simulink model "snb_b_ser2par"  (R2012b)
(part 2 of 57)

      |     current_names = current_names{1};
      |     numios = length(current_names);
      |     if length(current_widths) ~= numios,
      |         error('%d field names specified, but %d widths?', numios, length(current_widths));
      |     end
      | end
      | total_width = 0;
      | for ctr = 1 : length(current_widths),
      |     total_width = total_width + current_widths(ctr);
      | end
      | if total_width > 32,
      |     error('Total width must be 32 or less, set to %d.', total_width);
      | end
      mask Callback arith_types:
      | blk = gcb;
      | mode = get_param(blk, 'mode');
      | current_types = eval(get_param(blk, 'arith_types'));
      | numios = length(current_types);
      | if (strcmp(mode, 'one value') || strcmp(mode, 'fields of equal size')) && (length(current_types) > 1),
      |     error('Only one type may be specified for this mode.');
      | elseif strcmp(mode, 'fields of arbitrary size')
      |     current_names = textscan(strtrim(strrep(strrep(get_param(blk, 'names'), ']', ''), '[', '')), '%s');
      |     current_names = current_names{1};
      |     numios = length(current_names);
      |     if length(current_types) ~= numios,
      |         error('%d field names specified, but %d types?', numios, length(current_types));
      |     end
      | end
      | problem = 0;
      | for ctr = 1 : numios,
      |     t = current_types(ctr);
      |     if (t < 0) || (t > 2),
      |         problem = t;
      |         ctr = numios + 1;
      |     end
      | end
      | if problem ~= 0,
      |     error('Type cannot be %i, must be 0, 1 or 2.', problem);
      | end
      mask Callback bin_pts:
      | blk = gcb;
      | mode = get_param(blk, 'mode');
      | current_bins = eval(get_param(blk, 'bin_pts'));
      | if (strcmp(mode, 'one value') || strcmp(mode, 'fields of equal size')) && (length(current_bins) > 1),
      |     error('Only one binary pt may be specified for this mode.');
      | elseif strcmp(mode, 'fields of arbitrary size')
      |     current_names = textscan(strtrim(strrep(strrep(get_param(blk, 'names'), ']', ''), '[', '')), '%s');
      |     current_names = current_names{1};
      |     numios = length(current_names);
      |     if length(current_bins) ~= numios,
      |         error('%d field names specified, but %d binary pts?', numios, length(current_bins));
      |     end
      | end
  tmiss_p1 : Subsystem  Tag=xps:sw_reg  AncestorBlock=xps_library/software register  mask(swreg){mode=one value, io_dir=To Processor, io_delay=0, sample_period=1, names=reg, bitwidths=32, arith_types=0, bin_pts=0, sim_port=off, show_format=on}
      mask prompts: io_dir "I/O direction"; io_delay "I/O delay"; sample_period "Sample period"; names "Name:"; bitwidths "Bitwidth:"; arith_types "Type (ufix=0, fix=1, bool=2):"; bin_pts "Binary pt:"; sim_port "Provide sim input/output?"; show_format "Print format string?"
      mask init:
      | swreg_init(gcb)
      settings: AttributesFormatString=1output:uf32.0,
      mask TypeOptions mode: one value | fields of equal size | fields of arbitrary size
      mask Callback mode: swreg_cb(gcb);
      mask TypeOptions io_dir: To Processor | From Processor
      mask Callback io_dir:
      | mask_enables = get_param(gcb, 'MaskEnables');
      | mask_names = get_param(gcb, 'MaskNames');
      | if strcmp(get_param(gcb, 'io_dir'), 'To Processor'),
      |     mask_enables{ismember(mask_names, 'sample_period')} = 'off';
      | else
      |     mask_enables{ismember(mask_names, 'sample_period')} = 'on';
      | end
      | set_param(gcb, 'MaskEnables', mask_enables);
      mask Callback bitwidths:
      | blk = gcb;
      | mode = get_param(blk, 'mode');
      | current_widths = eval(get_param(blk, 'bitwidths'));
      | if (strcmp(mode, 'one value') || strcmp(mode, 'fields of equal size')) && (length(current_widths) > 1),
      |     error('Only one width may be specified for this mode.');
      | elseif strcmp(mode, 'fields of arbitrary size')
      |     current_names = textscan(strtrim(strrep(strrep(get_param(blk, 'names'), ']', ''), '[', '')), '%s');
      |     current_names = current_names{1};
      |     numios = length(current_names);
      |     if length(current_widths) ~= numios,
      |         error('%d field names specified, but %d widths?', numios, length(current_widths));
      |     end
      | end
      | total_width = 0;
      | for ctr = 1 : length(current_widths),
      |     total_width = total_width + current_widths(ctr);
      | end
      | if total_width > 32,
      |     error('Total width must be 32 or less, set to %d.', total_width);
      | end
      mask Callback arith_types:
      | blk = gcb;
      | mode = get_param(blk, 'mode');
      | current_types = eval(get_param(blk, 'arith_types'));
      | numios = length(current_types);
      | if (strcmp(mode, 'one value') || strcmp(mode, 'fields of equal size')) && (length(current_types) > 1),
      |     error('Only one type may be specified for this mode.');
      | elseif strcmp(mode, 'fields of arbitrary size')
      |     current_names = textscan(strtrim(strrep(strrep(get_param(blk, 'names'), ']', ''), '[', '')), '%s');
      |     current_names = current_names{1};
      |     numios = length(current_names);
      |     if length(current_types) ~= numios,
      |         error('%d field names specified, but %d types?', numios, length(current_types));
      |     end
      | end
      | problem = 0;
      | for ctr = 1 : numios,
      |     t = current_types(ctr);
      |     if (t < 0) || (t > 2),
      |         problem = t;
      |         ctr = numios + 1;
      |     end
      | end
      | if problem ~= 0,
      |     error('Type cannot be %i, must be 0, 1 or 2.', problem);
      | end
      mask Callback bin_pts:
      | blk = gcb;
      | mode = get_param(blk, 'mode');
      | current_bins = eval(get_param(blk, 'bin_pts'));
      | if (strcmp(mode, 'one value') || strcmp(mode, 'fields of equal size')) && (length(current_bins) > 1),
      |     error('Only one binary pt may be specified for this mode.');
      | elseif strcmp(mode, 'fields of arbitrary size')
      |     current_names = textscan(strtrim(strrep(strrep(get_param(blk, 'names'), ']', ''), '[', '')), '%s');
      |     current_names = current_names{1};
      |     numios = length(current_names);
      |     if length(current_bins) ~= numios,
      |         error('%d field names specified, but %d binary pts?', numios, length(current_bins));
      |     end
      | end
  trig0 : Subsystem  mask{mult_latency=3}
      mask prompts: mult_latency "Multiplier latency"
  trig1 : Subsystem  mask{mult_latency=3}
      mask prompts: mult_latency "Multiplier latency"
  trigger_level : Subsystem  Tag=xps:sw_reg  AncestorBlock=xps_library/software register  mask(swreg){mode=one value, io_dir=From Processor, io_delay=0, sample_period=1, names=trigger_level, bitwidths=32, arith_types=0, bin_pts=0, show_format=off}
      mask prompts: io_dir "I/O direction"; io_delay "I/O delay"; sample_period "Sample period"; names "Name:"; bitwidths "Bitwidth:"; arith_types "Type (ufix=0, fix=1, bool=2):"; bin_pts "Binary pt:"; show_format "Print format string?"
      mask init:
      | swreg_init(gcb)
      settings: AttributesFormatString=1input
      mask TypeOptions mode: one value | fields of equal size | fields of arbitrary size
      mask Callback mode: swreg_cb(gcb);
      mask TypeOptions io_dir: To Processor | From Processor
      mask Callback io_dir:
      | mask_enables = get_param(gcb, 'MaskEnables');
      | mask_names = get_param(gcb, 'MaskNames');
      | if strcmp(get_param(gcb, 'io_dir'), 'To Processor'),
      |     mask_enables{ismember(mask_names, 'sample_period')} = 'off';
      | else
      |     mask_enables{ismember(mask_names, 'sample_period')} = 'on';
      | end
      | set_param(gcb, 'MaskEnables', mask_enables);
      mask Callback bitwidths:
      | blk = gcb;
      | mode = get_param(blk, 'mode');
      | current_widths = eval(get_param(blk, 'bitwidths'));
      | if (strcmp(mode, 'one value') || strcmp(mode, 'fields of equal size')) && (length(current_widths) > 1),
      |     error('Only one width may be specified for this mode.');
      | elseif strcmp(mode, 'fields of arbitrary size')
      |     current_names = textscan(strtrim(strrep(strrep(get_param(blk, 'names'), ']', ''), '[', '')), '%s');
      |     current_names = current_names{1};
      |     numios = length(current_names);
      |     if length(current_widths) ~= numios,
      |         error('%d field names specified, but %d widths?', numios, length(current_widths));
      |     end
      | end
      | total_width = 0;
      | for ctr = 1 : length(current_widths),
      |     total_width = total_width + current_widths(ctr);
      | end
      | if total_width > 32,
      |     error('Total width must be 32 or less, set to %d.', total_width);
      | end
      mask Callback arith_types:
      | blk = gcb;
      | mode = get_param(blk, 'mode');
      | current_types = eval(get_param(blk, 'arith_types'));
      | numios = length(current_types);
      | if (strcmp(mode, 'one value') || strcmp(mode, 'fields of equal size')) && (length(current_types) > 1),
      |     error('Only one type may be specified for this mode.');
      | elseif strcmp(mode, 'fields of arbitrary size')
      |     current_names = textscan(strtrim(strrep(strrep(get_param(blk, 'names'), ']', ''), '[', '')), '%s');
      |     current_names = current_names{1};
      |     numios = length(current_names);
      |     if length(current_types) ~= numios,
      |         error('%d field names specified, but %d types?', numios, length(current_types));
      |     end
      | end
      | problem = 0;
      | for ctr = 1 : numios,
      |     t = current_types(ctr);
      |     if (t < 0) || (t > 2),
      |         problem = t;
      |         ctr = numios + 1;
      |     end
      | end
      | if problem ~= 0,
      |     error('Type cannot be %i, must be 0, 1 or 2.', problem);
      | end
      mask Callback bin_pts:
      | blk = gcb;
      | mode = get_param(blk, 'mode');
      | current_bins = eval(get_param(blk, 'bin_pts'));
      | if (strcmp(mode, 'one value') || strcmp(mode, 'fields of equal size')) && (length(current_bins) > 1),
      |     error('Only one binary pt may be specified for this mode.');
      | elseif strcmp(mode, 'fields of arbitrary size')
      |     current_names = textscan(strtrim(strrep(strrep(get_param(blk, 'names'), ']', ''), '[', '')), '%s');
      |     current_names = current_names{1};
      |     numios = length(current_names);
      |     if length(current_bins) ~= numios,
      |         error('%d field names specified, but %d binary pts?', numios, length(current_bins));
      |     end
      | end
  tx_metadata : Subsystem  Tag=xps:sw_reg  AncestorBlock=xps_library/software register  mask(swreg){mode=fields of arbitrary size, io_dir=From Processor, io_delay=0, sample_period=1, names=[porttx board_id], bitwidths=16, arith_types=0, bin_pts=0, sim_port=on, show_format=off}
      mask prompts: io_dir "I/O direction"; io_delay "I/O delay"; sample_period "Sample period"; names "Names [msb ... lsb]:"; bitwidths "Bitwidths [msb ... lsb]:"; arith_types "Types (ufix=0, fix=1, bool=2) [msb ... lsb]:"; bin_pts "Binary pts [msb ... lsb]:"; sim_port "Provide sim input/output?"; show_format "Print format string?"
      mask init:
      | swreg_init(gcb)
      settings: AttributesFormatString=2 inputs
      mask TypeOptions mode: one value | fields of equal size | fields of arbitrary size
      mask Callback mode: swreg_cb(gcb);
      mask TypeOptions io_dir: To Processor | From Processor
      mask Callback io_dir:
      | mask_enables = get_param(gcb, 'MaskEnables');
      | mask_names = get_param(gcb, 'MaskNames');
      | if strcmp(get_param(gcb, 'io_dir'), 'To Processor'),
      |     mask_enables{ismember(mask_names, 'sample_period')} = 'off';
      | else
      |     mask_enables{ismember(mask_names, 'sample_period')} = 'on';
      | end
      | set_param(gcb, 'MaskEnables', mask_enables);
      mask Callback bitwidths:
      | swreg_maskcheck(gcb);
      | % blk = gcb;
      | % mode = get_param(blk, 'mode');
      | % current_widths = eval(get_param(blk, 'bitwidths'));
      | % if (strcmp(mode, 'one value') || strcmp(mode, 'fields of equal size')) && (length(current_widths) > 1),
      | %     error('Only one width may be specified for this mode.');
      | % elseif strcmp(mode, 'fields of arbitrary size')
      | %     current_names = textscan(strtrim(strrep(strrep(get_param(blk, 'names'), ']', ''), '[', '')), '%s');
      | %     current_names = current_names{1};
      | %     numios = length(current_names);
      | %     if length(current_widths) ~= numios,
      | %         error('%d field names specified, but %d widths?', numios, length(current_widths));
      | %     end
      | % end
      | % total_width = 0;
      | % for ctr = 1 : length(current_widths),
      | %     total_width = total_width + current_widths(ctr);
      | % end
      | % if total_width > 32,
      | %     error('Total width must be 32 or less, set to %d.', total_width);
      | % end
      mask Callback arith_types:
      | [numios, ~, ~, ~, current_types] = swreg_maskcheck(gcb);
      | % blk = gcb;
      | % mode = get_param(blk, 'mode');
      | % current_types = eval(get_param(blk, 'arith_types'));
      | % numios = length(current_types);
      | % if (strcmp(mode, 'one value') || strcmp(mode, 'fields of equal size')) && (length(current_types) > 1),
      | %     error('Only one type may be specified for this mode.');
      | % elseif strcmp(mode, 'fields of arbitrary size')
      | %     current_names = textscan(strtrim(strrep(strrep(get_param(blk, 'names'), ']', ''), '[', '')), '%s');
      | %     current_names = current_names{1};
      | %     numios = length(current_names);
      | %     if length(current_types) ~= numios,
      | %         error('%d field names specified, but %d types?', numios, length(current_types));
      | %     end
      | % end
      | problem = 0;
      | for ctr = 1 : numios,
      |     t = current_types(ctr);
      |     if (t < 0) || (t > 2),
      |         problem = t;
      |         ctr = numios + 1;
      |     end
      | end
      | if problem ~= 0,
      |     error('Type cannot be %i, must be 0, 1 or 2.', problem);
      | end
      mask Callback bin_pts:
      | swreg_maskcheck(gcb);
      | % blk = gcb;
      | % mode = get_param(blk, 'mode');
      | % current_bins = eval(get_param(blk, 'bin_pts'));
      | % if (strcmp(mode, 'one value') || strcmp(mode, 'fields of equal size')) && (length(current_bins) > 1),
      | %     error('Only one binary pt may be specified for this mode.');
      | % elseif strcmp(mode, 'fields of arbitrary size')
      | %     current_names = textscan(strtrim(strrep(strrep(get_param(blk, 'names'), ']', ''), '[', '')), '%s');
      | %     current_names = current_names{1};
      | %     numios = length(current_names);
      | %     if length(current_bins) ~= numios,
      | %         error('%d field names specified, but %d binary pts?', numios, length(current_bins));
      | %     end
      | % end
  unpack_and_reorder : Subsystem  mask{n_bits_packet_size=9, n_bits_timestep=9+3, n_bits_fifo_depth=3, n_bits_buffer_depth=3, bram_latency=1}
      mask prompts: n_bits_packet_size "Packet size (2^? 80-bit words after unpacking)"; n_bits_timestep "Packet timestep (2^?)"; n_bits_fifo_depth "FIFO depth (2^? packets)"; n_bits_buffer_depth "Reorder buffer size (2^? packets)"; bram_latency "BRAM latency"
  up_debug : Subsystem  Tag=xps:sw_reg  AncestorBlock=xps_library/software register  mask(swreg){mode=one value, io_dir=From Processor, io_delay=0, sample_period=1, names=gbe_timestep, bitwidths=3, arith_types=0, bin_pts=0, sim_port=off, show_format=on}
      mask prompts: io_dir "I/O direction"; io_delay "I/O delay"; sample_period "Sample period"; names "Name:"; bitwidths "Bitwidth:"; arith_types "Type (ufix=0, fix=1, bool=2):"; bin_pts "Binary pt:"; sim_port "Provide sim input/output?"; show_format "Print format string?"
      mask init:
      | swreg_init(gcb)
      settings: AttributesFormatString=1input:uf3.0,
      mask TypeOptions mode: one value | fields of equal size | fields of arbitrary size
      mask Callback mode: swreg_cb(gcb);
      mask TypeOptions io_dir: To Processor | From Processor
      mask Callback io_dir:
      | mask_enables = get_param(gcb, 'MaskEnables');
      | mask_names = get_param(gcb, 'MaskNames');
      | if strcmp(get_param(gcb, 'io_dir'), 'To Processor'),
      |     mask_enables{ismember(mask_names, 'sample_period')} = 'off';
      | else
      |     mask_enables{ismember(mask_names, 'sample_period')} = 'on';
      | end
      | set_param(gcb, 'MaskEnables', mask_enables);
      mask Callback bitwidths:
      | blk = gcb;
      | mode = get_param(blk, 'mode');
      | current_widths = eval(get_param(blk, 'bitwidths'));
      | if (strcmp(mode, 'one value') || strcmp(mode, 'fields of equal size')) && (length(current_widths) > 1),
      |     error('Only one width may be specified for this mode.');
      | elseif strcmp(mode, 'fields of arbitrary size')
      |     current_names = textscan(strtrim(strrep(strrep(get_param(blk, 'names'), ']', ''), '[', '')), '%s');
      |     current_names = current_names{1};
      |     numios = length(current_names);
      |     if length(current_widths) ~= numios,
      |         error('%d field names specified, but %d widths?', numios, length(current_widths));
      |     end
      | end
      | total_width = 0;
      | for ctr = 1 : length(current_widths),
      |     total_width = total_width + current_widths(ctr);
      | end
      | if total_width > 32,
      |     error('Total width must be 32 or less, set to %d.', total_width);
      | end
      mask Callback arith_types:
      | blk = gcb;
      | mode = get_param(blk, 'mode');
      | current_types = eval(get_param(blk, 'arith_types'));
      | numios = length(current_types);
      | if (strcmp(mode, 'one value') || strcmp(mode, 'fields of equal size')) && (length(current_types) > 1),
      |     error('Only one type may be specified for this mode.');
      | elseif strcmp(mode, 'fields of arbitrary size')
      |     current_names = textscan(strtrim(strrep(strrep(get_param(blk, 'names'), ']', ''), '[', '')), '%s');
      |     current_names = current_names{1};
      |     numios = length(current_names);
      |     if length(current_types) ~= numios,
      |         error('%d field names specified, but %d types?', numios, length(current_types));
      |     end
      | end
      | problem = 0;
      | for ctr = 1 : numios,
      |     t = current_types(ctr);
      |     if (t < 0) || (t > 2),
      |         problem = t;
      |         ctr = numios + 1;
      |     end
      | end
      | if problem ~= 0,
      |     error('Type cannot be %i, must be 0, 1 or 2.', problem);
      | end
      mask Callback bin_pts:
      | blk = gcb;
      | mode = get_param(blk, 'mode');
      | current_bins = eval(get_param(blk, 'bin_pts'));
      | if (strcmp(mode, 'one value') || strcmp(mode, 'fields of equal size')) && (length(current_bins) > 1),
      |     error('Only one binary pt may be specified for this mode.');
      | elseif strcmp(mode, 'fields of arbitrary size')
      |     current_names = textscan(strtrim(strrep(strrep(get_param(blk, 'names'), ']', ''), '[', '')), '%s');
      |     current_names = current_names{1};
      |     numios = length(current_names);
      |     if length(current_bins) ~= numios,
      |         error('%d field names specified, but %d binary pts?', numios, length(current_bins));
      |     end
      | end
  updebug : Subsystem
      mask Display: fprintf('UP\nDEBUG')
  xps : xps_library/XSG core config  Tag=xps:xsg  hw_sys=ROACH2:sx475t  clk_src=sys_clk  ROACH_clk_src=adc0_clk  ROACH2_clk_src=sys_clk  MKDIG_clk_src=sys_clk  clk_rate=228  sample_period=1  synthesis_tool=XST
  tag scope: cnt_rst=global, gbe_timestep=global, up_cnt_rst=global, wintime_snap_wesel=global
  wires:
  gbe0/1(led_up) -> Inverter/1, [up_gbe0]
  gbe0/2(led_rx) -> [rx_gbe0]
  gbe0/3(led_tx) -> [tx_gbe0]
  gbe0/5(tx_overflow) -> [tx_over_gbe0], [of_xaui0]
  gbe0/12(rx_overrun) -> [rxover_gbe0]
  gbe0/11(rx_bad_frame) -> [rxbad_gbe0]
  gbe0/6(rx_data) -> [rxdata_gbe0]
  gbe0/7(rx_valid) -> [rxvld_gbe0]
  gbe0/8(rx_source_ip) -> [rxip_gbe0]
  gbe0/9(rx_source_port) -> [rxport_gbe0]
  gbe0/10(rx_end_of_frame) -> [rxeof_gbe0]
  Inverter/1 -> [ldn_xaui0]
  [gbe_rst] -> Delay12/1
  gbe1/1(led_up) -> [up_gbe1], Inverter1/1
  gbe1/2(led_rx) -> [rx_gbe1]
  gbe1/3(led_tx) -> [tx_gbe1]
  gbe1/4(tx_afull) -> [tx_full_gbe1]
  gbe1/5(tx_overflow) -> [tx_over_gbe1], [of_xaui1]
  gbe1/12(rx_overrun) -> [rxover_gbe1]
  gbe1/11(rx_bad_frame) -> [rxbad_gbe1]
  gbe1/6(rx_data) -> [rxdata_gbe1]
  gbe1/7(rx_valid) -> [rxvld_gbe1]
  gbe1/8(rx_source_ip) -> [rxip_gbe1]
  gbe1/9(rx_source_port) -> [rxport_gbe1]
  gbe1/10(rx_end_of_frame) -> [rxeof_gbe1]
  Inverter1/1 -> [ldn_xaui1]
  Delay12/1 -> gbe1/1(rst)
  gbe2/1(led_up) -> [up_gbe2], Inverter3/1
  gbe2/2(led_rx) -> [rx_gbe2]
  gbe2/3(led_tx) -> [tx_gbe2]
  gbe2/4(tx_afull) -> [tx_full_gbe2]
  gbe2/5(tx_overflow) -> [tx_over_gbe2], [of_xaui2]
  gbe2/12(rx_overrun) -> [rxover_gbe2]
  gbe2/11(rx_bad_frame) -> [rxbad_gbe2]
  gbe2/6(rx_data) -> [rxdata_gbe2]
  gbe2/7(rx_valid) -> [rxvld_gbe2]
  gbe2/8(rx_source_ip) -> [rxip_gbe2]
  gbe2/9(rx_source_port) -> [rxport_gbe2]
  gbe2/10(rx_end_of_frame) -> [rxeof_gbe2]
  Inverter3/1 -> [ldn_xaui2]
  gbe3/1(led_up) -> [up_gbe3], Inverter4/1
  gbe3/2(led_rx) -> [rx_gbe3]
  gbe3/3(led_tx) -> [tx_gbe3]
  gbe3/4(tx_afull) -> [tx_full_gbe3]
  gbe3/5(tx_overflow) -> [tx_over_gbe3], [of_xaui3]
  gbe3/12(rx_overrun) -> [rxover_gbe3]
  gbe3/11(rx_bad_frame) -> [rxbad_gbe3]
  gbe3/6(rx_data) -> [rxdata_gbe3]
  gbe3/7(rx_valid) -> [rxvld_gbe3]
  gbe3/8(rx_source_ip) -> [rxip_gbe3]
  gbe3/9(rx_source_port) -> [rxport_gbe3]
  gbe3/10(rx_end_of_frame) -> [rxeof_gbe3]
  Inverter4/1 -> [ldn_xaui3]
  gbe0/4(tx_afull) -> [tx_full_gbe0]
  bus_expand1/2(lsb_out1) -> aligned/2, misaligned/2
  bus_expand1/1(msb_out2) -> misaligned/1, aligned/1
  aligned/1 -> Register4/1
  misaligned/1 -> Register5/1
  [clr_status] -> Register5/2, Register4/2
  Register5/1 -> [data_misaligned]
  Register4/1 -> [data_aligned]
  edge_detect3/1(out) -> pipeline4/1(d)
  edge_detect4/1(out) -> pipeline3/1(d)
  edge_detect5/1(out) -> pipeline2/1(d)
  [unpack_en] -> Register5/3, Register4/3
  [unpack_recvd] -> bus_expand1/1(bus_in)
  Delay8/1 -> [unpack_d80]
  Delay59/1 -> [unpack_en]  "re80_v"
  Delay62/1 -> aligned1/1
  Delay71/1 -> aligned1/2
  Delay78/1 -> [unpack_recvd]
  [sys_rst] -> edge_detect9/1(in)
  [rxdata_gbe0] -> concat0/1
  [rxdata_gbe1] -> concat0/2
  [rxdata_gbe2] -> concat0/3
  [rxdata_gbe3] -> concat0/4
  [rxeof_gbe0] -> concat1/1
  [rxeof_gbe1] -> concat1/2
  [rxeof_gbe2] -> concat1/3
  [rxeof_gbe3] -> concat1/4
  [rxvld_gbe0] -> concat3/1
  [rxvld_gbe1] -> concat3/2
  [rxvld_gbe2] -> concat3/3
  [rxvld_gbe3] -> concat3/4
  bus_expand2/1(msb_out2) -> Delay62/1
  bus_expand2/2(lsb_out1) -> Delay71/1
  control/2(in_arm) -> edge_detect5/1(in)
  Delay82/1 -> [unpack_timestamp]  "tstamp"
  control/13(in_cnt_rst) -> edge_detect1/1(in)
  concat0/1 -> Delay30/1
  concat1/1 -> Delay31/1
  concat3/1 -> Delay32/1
  constant/1 -> unpack_and_reorder/5(transmit)
  unpack_and_reorder/4(timestamp) -> Delay82/1
  unpack_and_reorder/5(recvd) -> Delay78/1
  unpack_and_reorder/6(of_count) -> bus_expand2/1(bus_in)
  unpack_and_reorder/1(sync) -> Delay41/1
  unpack_and_reorder/7(fifo_of) -> [unpack_fifo_or]
  edge_detect1/1(out) -> pipeline14/1(d)
  control/4(in_gbe_rst) -> pipeline5/1(d)
  control/1(in_sys_rst) -> pipeline/1(d)
  Constant4/1 -> gbe1/8(rx_overrun_ack), gbe1/7(rx_ack)
  [gbe_rst] -> Delay10/1
  Delay10/1 -> gbe2/1(rst)
  Constant23/1 -> gbe2/8(rx_overrun_ack), gbe2/7(rx_ack)
  [gbe_rst] -> Delay11/1
  Delay11/1 -> gbe3/1(rst)
  Constant33/1 -> gbe3/8(rx_overrun_ack), gbe3/7(rx_ack)
  [gbe_rst] -> Delay14/1
  [s64_d0] -> Delay24/1
  [s64_ip] -> Delay25/1
  [s64_port] -> Delay26/1
  Logical2/1 -> gbe0/3(tx_valid)
  Constant20/1 -> gbe0/8(rx_overrun_ack), gbe0/7(rx_ack)
  [gbe_cnt_rst] -> Delay47/1
  [gbe_cnt_rst] -> Delay46/1
  [gbe_cnt_rst] -> Delay45/1
  [gbe_cnt_rst] -> Delay44/1
  [gbe_txen] -> Logical4/2, Logical2/2
  [s64_v0] -> Logical2/1
  [s64_d1] -> Delay27/1
  [s64_ip] -> Delay28/1
  [s64_port] -> Delay33/1
  [gbe_txen] -> Logical3/2, Logical7/2
  [s64_v1] -> Logical7/1
  Logical7/1 -> gbe1/3(tx_valid)
  [s64_d2] -> Delay35/1
  [s64_ip] -> Delay36/1
  [s64_port] -> Delay37/1
  [gbe_txen] -> Logical11/2, Logical8/2
  [s64_v2] -> Logical8/1
  [s64_d3] -> Delay38/1
  [s64_ip] -> Delay39/1
  [s64_port] -> Delay40/1
  [gbe_txen] -> Logical12/2, Logical9/2
  [s64_v3] -> Logical9/1
  Logical8/1 -> gbe2/3(tx_valid)
  Logical9/1 -> gbe3/3(tx_valid)
  Constant10/1 -> iptx_base/1(sim_1)
  iptx_base/1(in_reg) -> Delay20/1
  Constant3/1 -> tx_metadata/1(sim_1)
  tx_metadata/2(in_board_id) -> Delay22/1
  Constant5/1 -> tx_metadata/2(sim_2)
  pipeline/1(q) -> [sys_rst]
  pipeline2/1(q) -> [arm]
  pipeline3/1(q) -> [clr_status]
  pipeline4/1(q) -> [clr_adc_bad]
  pipeline5/1(q) -> [gbe_rst]
  pipeline6/1(q) -> [gbe_txen]
  pipeline8/1(q) -> [adc_protect_disable]
  pipeline9/1(q) -> [tvg_en]
  pipeline10/1(q) -> [ct_tvg]
  pipeline11/1(q) -> [packetiser_tvg]
  pipeline12/1(q) -> [fd_fs_tvg]
  pipeline13/1(q) -> [tvg_adc_en]
  pipeline14/1(q) -> [cnt_rst]
  control/12(in_tvg_adc) -> pipeline13/1(d)
  tx_metadata/1(in_porttx) -> Delay21/1
  unpack_and_reorder/8(packet_of) -> [fifo_pktof]
  Delay29/1 -> unpack_and_reorder/1(rst)
  Delay30/1 -> unpack_and_reorder/2(din)
  Delay31/1 -> unpack_and_reorder/3(eof)
  Delay32/1 -> unpack_and_reorder/4(en)
  Delay44/1 -> gbe3/9(debug_rst)
  Delay45/1 -> gbe2/9(debug_rst)
  Delay46/1 -> gbe1/9(debug_rst)
  Delay47/1 -> gbe0/9(debug_rst)
  edge_detect2/1(out) -> pipeline7/1(d)
  pipeline7/1(q) -> [gbe_cnt_rst]
  control/14(in_gbe_cnt_rst) -> edge_detect2/1(in)
  Logical3/1 -> gbe1/6(tx_end_of_frame)
  [s64_eof1] -> Logical3/1
  Logical4/1 -> gbe0/6(tx_end_of_frame)
  [s64_eof0] -> Logical4/1
  Logical11/1 -> gbe2/6(tx_end_of_frame)
  [s64_eof2] -> Logical11/1
  Logical12/1 -> gbe3/6(tx_end_of_frame)
  [s64_eof3] -> Logical12/1
  Delay14/1 -> gbe0/1(rst)
  edge_detect7/1(out) -> pipeline15/1(d)
  pipeline15/1(q) -> [up_cnt_rst]
  Delay20/1 -> [tx_ip_base]
  Delay21/1 -> [tx_port]
  Delay22/1 -> [tx_board_id]
  Delay24/1 -> gbe0/2(tx_data)
  Delay25/1 -> gbe0/4(tx_dest_ip)
  Delay26/1 -> gbe0/5(tx_dest_port)
  Delay27/1 -> gbe1/2(tx_data)
  Delay28/1 -> gbe1/4(tx_dest_ip)
  Delay33/1 -> gbe1/5(tx_dest_port)
  Delay35/1 -> gbe2/2(tx_data)
  Delay36/1 -> gbe2/4(tx_dest_ip)
  Delay37/1 -> gbe2/5(tx_dest_port)
  Delay38/1 -> gbe3/2(tx_data)
  Delay39/1 -> gbe3/4(tx_dest_ip)
  Delay40/1 -> gbe3/5(tx_dest_port)
  unpack_and_reorder/2(dout) -> Delay8/1
  unpack_and_reorder/3(dvalid) -> Delay59/1
  unpack_and_reorder/9(spead_error) -> Terminator1/1
  unpack_and_reorder/10(discarding) -> Terminator2/1
  unpack_and_reorder/11(timestep_error) -> [timestep_error]
  Constant25/1 -> trigger_level/1(sim_1)
  [d80_adc1] -> trig1/2(adc_data)
  trig1/3(trig) -> [trans_stop_1]
  trig1/2(data) -> [trans_d80_1]
  trig0/2(data) -> [trans_d80_0]
  trig0/3(trig) -> [trans_stop_0]
  [d80_adc0] -> trig0/2(adc_data)
  trig1/1(synco) -> [trans_valid80]
  [sync80] -> Concat6/1
  [time80] -> Slice14/1
  Concat6/1 -> trig0/1(synci)
  trig0/1(synco) -> bus_expand/1(bus_in)
  bus_expand/1(msb_out2) -> [trans_trig]
  Slice14/1 -> Concat6/2
  bus_expand/2(lsb_out1) -> [trans_time]
  [valid80] -> trig1/1(synci)
  trigger_level/1(in_trigger_level) -> pipeline17/1(d)
  [unpack_en] -> en_gen/2(en)
  [unpack_timestamp] -> en_gen/3(time_in)
  en_gen/1(dout) -> sync_gen/1(din)
  sync_gen/1(sync) -> data_tvg1/2(sync_in), data_tvg0/2(sync_in)
  data_tvg0/3(dvalid) -> [valid80]
  data_tvg0/1(sync_out) -> [sync80]
  bus_expand6/2(lsb_out1) -> data_tvg1/3(din)
  data_tvg0/2(dout) -> [d80_adc0]
  [tvg_d80_en] -> en_gen/5(tvg_en)
  pipeline17/1(q) -> trig1/3(trig_pnt), trig0/3(trig_pnt)
  [unpack_d80] -> en_gen/1(din)
  bus_expand6/1(msb_out2) -> data_tvg0/3(din)
  data_tvg0/4(misco) -> [time80]
  sync_gen/5(misco) -> data_tvg1/5(misci)
  data_tvg1/2(dout) -> [d80_adc1]
  data_tvg1/3(dvalid) -> Terminator9/1
  data_tvg1/1(sync_out) -> Terminator4/1
  Concat/1 -> en_gen/4(misci)
  [unpack_adc_or] -> Concat/1
  [data_misaligned] -> Concat/2
  data_tvg1/4(misco) -> bus_expand19/1(bus_in)
  bus_expand19/1(msb_out2) -> [adc_or_flag]
  bus_expand19/2(lsb_out1) -> [missing_flag]
  [tvg_adc_en] -> data_tvg0/1(tvg_en), data_tvg1/1(tvg_en)
  en_gen/3(time_out) -> sync_gen/3(time_in)
  en_gen/2(dvalid) -> sync_gen/2(en)
  en_gen/4(misco) -> Slice20/1, Slice19/1
  Slice19/1 -> sync_gen/4(misci)
  Slice20/1 -> sync_gen/5(relock)
  sync_gen/4(time_out) -> data_tvg0/5(misci)
  sync_gen/2(dout) -> bus_expand6/1(bus_in)
  sync_gen/3(dvalid) -> data_tvg1/4(en), data_tvg0/4(en)
  [timestep_error] -> Concat/3
  Slice/1 -> pipeline16/1(d)
  pipeline16/1(q) -> local_time_lsw/1(out_timestamp_lsw)
  Slice16/1 -> Convert1/1
  pipeline47/1(q) -> local_time_msw/1(out_timestamp_msw)
  Convert1/1 -> pipeline47/1(d)
  Concat2/1 -> Slice16/1, [time80_48], Slice/1
  [time80] -> Concat2/1
  Constant53/1 -> Concat2/2
  control/15(in_unpack_cnt_rst) -> edge_detect7/1(in)
  pipeline18/1(q) -> [snappfb_arm]
  control/17(in_snappfb_arm) -> pipeline18/1(d)
  control/5(in_gbe_txen) -> pipeline6/1(d)
  control/6(in_adc_bad_clr) -> edge_detect3/1(in)
  control/7(in_adc_protect_disable) -> pipeline8/1(d)
  control/8(in_tvg_en) -> pipeline9/1(d)
  control/9(in_tvg_ct) -> pipeline10/1(d)
  control/10(in_tvg_packetiser) -> pipeline11/1(d)
  control/11(in_tvg_fdfs) -> pipeline12/1(d)
  pipeline19/1(q) -> [tvg_d80_en]
  control/20(in_tvg_d80) -> pipeline19/1(d)
  aligned1/1 -> [unpack_adc_or]
  control/3(in_status_clr) -> edge_detect4/1(in)
  Delay41/1 -> [unpack_sync]
  Register11/1 -> Slice9/1, Slice7/1
  [time80] -> pipeline54/1(d)
  Slice7/1 -> sync_timestamp_msw/1(out_reg)
  [sync80] -> pipeline52/1(d)
  [valid80] -> pipeline53/1(d)
  Register12/1 -> Logical1/1  "armed"
  Logical1/1 -> Register12/2, Register11/2
  pipeline52/1(q) -> Register12/3, Register12/1
  pipeline53/1(q) -> Logical1/2
  pipeline54/1(q) -> Register11/1
  [valid80] -> pipeline55/1(d)
  pipeline55/1(q) -> Delay42/1, edge_detect13/1(in)
  counter8/1 -> Register13/1
  edge_detect13/1(out) -> counter8/1, Register13/2
  Delay42/1 -> counter8/2
  Slice9/1 -> sync_timestamp_lsw/1(out_time_lsw)
  Register13/1 -> sync_timestamp_lsw/2(out_pkt_size)
  pipeline56/1(q) -> edge_detect14/1(in)
  edge_detect14/1(out) -> counter9/2
  [timestep_error] -> pipeline56/1(d)
  [cnt_rst] -> pipeline57/1(d)
  pipeline57/1(q) -> counter9/1
  pipeline58/1(q) -> edge_detect15/1(in)
  edge_detect15/1(out) -> counter10/2
  [sync80] -> pipeline58/1(d)
  [cnt_rst] -> pipeline51/1(d)
  pipeline51/1(q) -> counter10/1
  pipeline59/1(q) -> edge_detect16/1(in)
  edge_detect16/1(out) -> counter11/2
  [valid80] -> pipeline59/1(d)
  [cnt_rst] -> pipeline60/1(d)
  pipeline60/1(q) -> counter11/1
  counter9/1 -> sync_timestamp_lsw/3(out_tstep_err_ctr)
  counter10/1 -> sync_timestamp_lsw/4(out_sync80_ctr)
  counter11/1 -> sync_timestamp_lsw/5(out_valid80_ctr)
  pipeline48/1(q) -> [wintime_snap_wesel]
  control/21(in_wintime_snap_wesel) -> pipeline48/1(d)
  edge_detect9/1(out) -> Delay29/1
  [up_p0_missed_time_ctr] -> Delay76/1(d)
  [up_p1_missed_time_ctr] -> Delay77/1(d)
  [up_p0_missed_time] -> Delay81/1(d)
  [up_p1_missed_time] -> Delay83/1(d)
  Delay81/1(q) -> Slice10/1
  Delay83/1(q) -> Slice11/1
  Delay76/1(q) -> tmiss_ctr/1(out_p0)
  Delay77/1(q) -> tmiss_ctr/2(out_p1)
  [unpack_recvd] -> Slice17/1, Slice12/1
  Inverter2/1 -> Logical5/1
  [unpack_en] -> Logical6/2, Logical5/2
  Logical5/1 -> counter20/2
  [cnt_rst] -> Delay79/1(d)
  counter20/1 -> recverr_ctr/1(out_p0)
  counter21/1 -> mcnt_relock/1(out_reg)
  [mcnt_relock] -> counter21/2
  Slice10/1 -> tmiss_p0/1(out_reg)
  Slice11/1 -> tmiss_p1/1(out_reg)
  counter22/1 -> recverr_ctr/2(out_p1)
  Slice12/1 -> Inverter2/1
  Logical6/1 -> counter22/2
  Slice17/1 -> Inverter5/1
  Inverter5/1 -> Logical6/1
  [up_timestep_error_future] -> counter23/2
  [up_timestep_error_past] -> counter13/2
  Delay79/1(q) -> counter22/1, counter23/1, counter13/1, counter21/1, counter20/1
  counter23/1 -> timestep_ages/1(out_future)
  counter13/1 -> timestep_ages/2(out_past)
  pipeline67/1(q) -> [snappfb_dsel]
  control/18(in_snappfb_dsel) -> pipeline67/1(d)
  pipeline72/1(q) -> [snapcoarse_arm]
  control/16(in_snapcoarse_arm) -> pipeline72/1(d)
  pipeline77/1(q) -> [snapquant_arm]
  control/19(in_snapquant_arm) -> pipeline77/1(d)
  [up_gbe0] -> gbe_status/1(out_gbe0_linkup)
  [up_gbe1] -> gbe_status/2(out_gbe1_linkup)
  [up_gbe2] -> gbe_status/3(out_gbe2_linkup)
  [up_gbe3] -> gbe_status/4(out_gbe3_linkup)
  up_debug/1(in_gbe_timestep) -> Delay88/1(d)
  Delay88/1(q) -> [gbe_timestep]
  unpack_and_reorder/12(mcnt_relock) -> [mcnt_relock]
  Constant1/1 -> [s64_d0]
  Constant2/1 -> [s64_v0]
  Constant6/1 -> [s64_d1]
  Constant7/1 -> [s64_v1]
  Constant8/1 -> [s64_ip]
  Constant9/1 -> [s64_port]
  Constant11/1 -> [s64_d2]
  Constant12/1 -> [s64_v2]
  Constant13/1 -> [s64_d3]
  Constant14/1 -> [s64_v3]
  Constant15/1 -> [s64_eof1]
  Constant17/1 -> [s64_eof0]
  Constant16/1 -> [s64_eof2]
  Constant18/1 -> [s64_eof3]
  Constant21/1 -> snap_mixed0/4(trig)
  bus_expand7/1(msb_out2) -> snap_mixed0/1(in_p0_18r)  "indata_r"
  bus_expand7/2(lsb_out1) -> snap_mixed0/2(in_p0_18i)  "in_data_i"
  pfb_fft/1(sync_out) -> Delay15/1
  pfb_fft/2(dv_out) -> Delay16/1
  pfb_fft/3(pol0_out) -> Delay17/1
  pfb_fft/4(pol1_out) -> Delay18/1
  Delay15/1 -> serial_to_4par1/1(sync), serial_to_4par/1(sync)
  Delay16/1 -> snap_pfb0/4(we), snap_pfb0/3(in_dv), serial_to_4par1/2(dv), serial_to_4par/2(dv)
  Delay17/1 -> bus_expand4/1(bus_in), serial_to_4par/3(data)
  Delay18/1 -> serial_to_4par1/3(data)
  Delay2/1 -> pfb_fft/1(sync)
  Delay3/1 -> pfb_fft/2(dv)
  Delay4/1 -> pfb_fft/3(pol0)
  Delay5/1 -> pfb_fft/4(pol1)
  serial_to_4par1/1(sync_out) -> Terminator5/1
  serial_to_4par1/2(dv_out) -> Terminator3/1
  serial_to_4par1/3(data0_old) -> Terminator6/1
  serial_to_4par1/4(data1) -> Terminator7/1
  serial_to_4par1/5(data2) -> Terminator8/1
  serial_to_4par1/6(data3_new) -> Terminator10/1
  serial_to_4par/1(sync_out) -> Delay6/1
  serial_to_4par/2(dv_out) -> Delay7/1
  serial_to_4par/3(data0_old) -> Delay9/1
  serial_to_4par/4(data1) -> Delay13/1
  serial_to_4par/5(data2) -> Delay19/1
  serial_to_4par/6(data3_new) -> Delay23/1
  Register/1 -> Logical10/2
  Logical10/1 -> Register/2, snap_serial0/9(trig), snap_serial1/5(trig)
  bus_expand3/1(msb_out2) -> snap_serial0/1(in_d0_r)
  bus_expand3/2(lsb_out1) -> snap_serial0/2(in_d0_i)
  bus_expand5/2(lsb_out1) -> snap_serial0/4(in_d1_i)
  bus_expand5/1(msb_out2) -> snap_serial0/3(in_d1_r)
  Delay7/1 -> snap_serial1/4(we), snap_serial1/3(in_dv), snap_serial0/8(we), snap_serial0/7(in_dv)
  Delay9/1 -> bus_expand3/1(bus_in)
  Delay13/1 -> bus_expand5/1(bus_in)
  Delay19/1 -> bus_expand8/1(bus_in)
  Delay23/1 -> bus_expand9/1(bus_in)
  snaparm/1(in_sersnap_arm) -> edge_detect/1(in)
  edge_detect/1(out) -> Register/1, Register/3
  filter/3(Out3) -> snap_mixed0/3(we), Delay3/1
  filter/2(Out2) -> bus_expand7/1(bus_in), Delay5/1, Delay4/1
  [valid80] -> Delay34/1
  [sync80] -> Delay1/1
  [d80_adc0] -> Delay43/1
  filter/1(Out1) -> Delay2/1
  Delay1/1 -> filter/1(sync)
  Delay34/1 -> filter/2(dv)
  Delay43/1 -> filter/3(data)
  pfb_fft/5(spec_sync) -> Delay49/1
  Delay49/1 -> Delay48/1, snap_pfb0/5(trig)
  Delay48/1 -> Delay50/1
  Delay50/1 -> Logical10/1
  bus_expand4/2(lsb_out1) -> snap_pfb0/2(in_p0_18i)
  bus_expand4/1(msb_out2) -> snap_pfb0/1(in_p0_18r)
  bus_expand8/2(lsb_out1) -> snap_serial0/6(in_d2_i)
  bus_expand8/1(msb_out2) -> snap_serial0/5(in_d2_r)
  bus_expand9/1(msb_out2) -> snap_serial1/1(in_d3_r)
  bus_expand9/2(lsb_out1) -> snap_serial1/2(in_d3_i)
